simulink library "Lib_Turbo_FlowPathChar_TMATS"  (R2012b)
settings: Solver=ode45  StartTime=0.0  StopTime=10.0  RelTol=1e-3
Description:
  | Thomas Modules
settings Model: Creator=jwchapm2  LastModifiedBy=jwchapm2

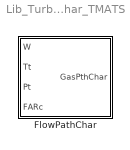
== system Lib_Turbo_FlowPathChar_TMATS ==
  FlowPathChar : Subsystem  mask(T-MATS: Flow Path Characteristics Library Block){}
      mask help: This block creates a flow path characteristics bus for input into the system.
      mask Help: web(which('Turbo_TMATS_FPC.html'),'-helpbrowser')

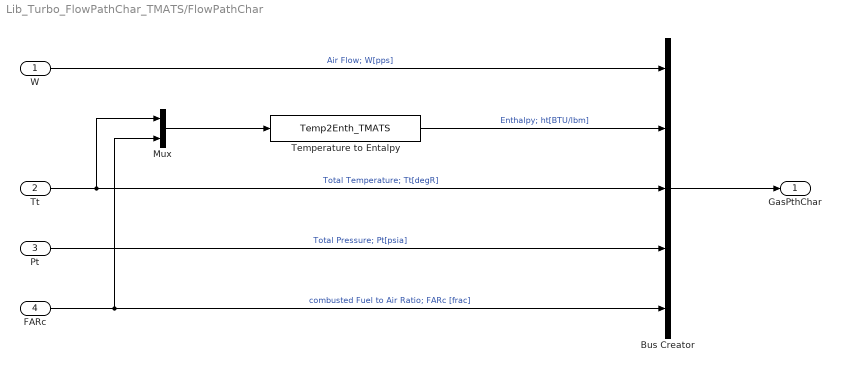
== system Lib_Turbo_FlowPathChar_TMATS/FlowPathChar ==
  W : Inport
  Tt : Inport  Port=2
  Pt : Inport  Port=3
  FARc : Inport  Port=4
  Bus Creator : BusCreator  Inputs=5
  Mux : Mux  Inputs=2
  Temperature to Entalpy : S-Function  FunctionName=Temp2Enth_TMATS  EnableBusSupport=off
  GasPthChar : Outport
  wires:
  W/1 -> Bus Creator/1  "Air Flow; W[pps]"
  Pt/1 -> Bus Creator/4  "Total Pressure; Pt[psia]"
  FARc/1 -> Mux/2, Bus Creator/5  "combusted Fuel to Air Ratio; FARc [frac]"
  Bus Creator/1 -> GasPthChar/1
  Tt/1 -> Mux/1, Bus Creator/3  "Total Temperature; Tt[degR]"
  Temperature to Entalpy/1 -> Bus Creator/2  "Enthalpy; ht[BTU/lbm]"
  Mux/1 -> Temperature to Entalpy/1
